simulink model "test"  (R2017b)
settings: Solver=FixedStepAuto  StartTime=0.0  StopTime=Tend  RelTol=1e-3  EnableMultiTasking=on
StartFcn:
  | params
values from neighbouring files (symbols this model uses):
  Tend = 30    [params.m]    (also in readingVoltage.m = 10)
  Ts = 0.01    [params.m]    (also in readingVoltage.m = 0.1)
libraries: arduinolib x4, cstblocks x1
settings Model: SimulationMode=external  ExtModeTrigDuration=2  Creator=s-tsujii  LastModifiedBy=s-tsujii
settings OptimizationCC: PassReuseOutputArgsThreshold=0  MaxStackSize=64
settings DebuggingCC: ParameterTunabilityLossMsg=error
settings HardwareCC: ProdBitPerInt=16  ProdBitPerPointer=16  ProdBitPerSizeT=16  ProdBitPerPtrDiffT=16  ProdLargestAtomicFloat=None  ProdWordSize=8  ProdHWDeviceType=Atmel->AVR  UseEmbeddedCoderFeatures=off  UseSimulinkCoderFeatures=off
settings SFSimCC: MATLABDynamicMemAlloc=off
settings RTWCC: SystemTargetFile=ert.tlc  HardwareBoard=Arduino Uno  TLCOptions=-aInlineSetEventsForThisBaseRateFcn=TLC_FALSE -aSuppressMultiTaskScheduler=TLC_FALSE -aRateBasedStepFcn=1  TemplateMakefile=ert_default_tmf  GenerateReport=on  Toolchain=Arduino AVR  BuildConfiguration=Faster Runs  LaunchReport=on
settings CodeAppCC: ForceParamTrailComments=on  OperatorAnnotations=on  MangleLength=10
settings ERTTargetCC: ERTCustomFileBanners=off  SupportContinuousTime=on  SupportNonInlinedSFcns=on  RemoveResetFunc=off  SupportVariableSizeSignals=on  ModelStepFunctionPrototypeControlCompliant=off

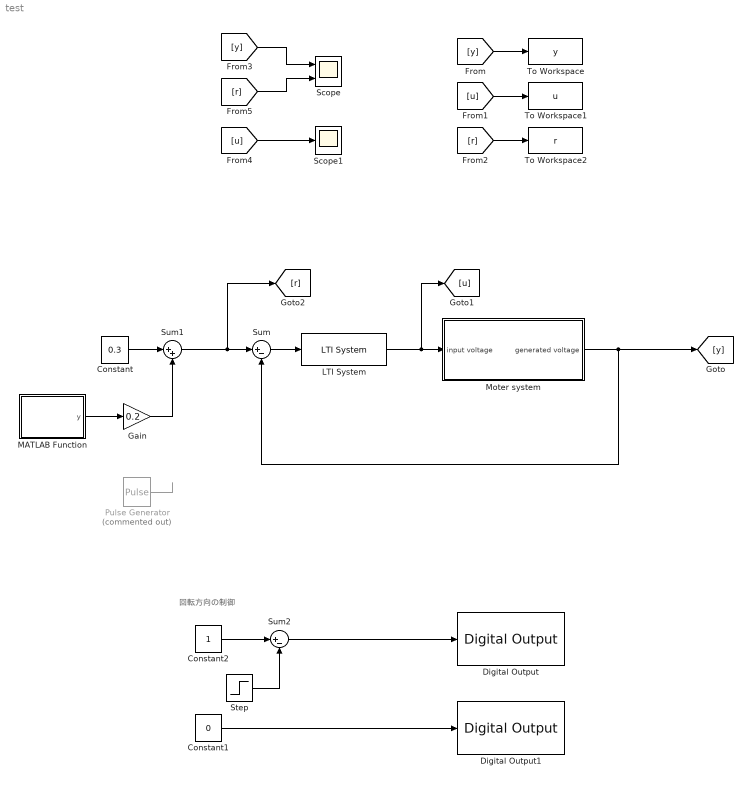
== system test ==
  note: 回転方向の制御
  Constant : Constant  Value=0.3
  Constant1 : Constant  Value=0
  Constant2 : Constant
  Digital Output : arduinolib/Digital Output  pinNumber=6  blockPlatform=arduino
  Digital Output1 : arduinolib/Digital Output  pinNumber=7  blockPlatform=arduino
  Gain : Gain  Gain=0.2
  LTI System : cstblocks/LTI System  sys=Cfb  IC=[]
  MATLAB Function : MATLAB Function  TreatAsAtomicUnit=on
  Moter system : Subsystem
  Pulse Generator : DiscretePulseGenerator  Commented=on  Amplitude=0.5  Period=4/Ts  PulseWidth=0.5*4/Ts  SampleTime=Ts
  Scope : Scope  NumInputPorts=2
  Scope1 : Scope
  Step : Step  Time=Tend-Ts  SampleTime=Ts
  Sum : Sum  Inputs=|+-
  Sum1 : Sum  Inputs=|++
  Sum2 : Sum  Inputs=|+-
  To Workspace : ToWorkspace  VariableName=y  SaveFormat=Structure With Time  SampleTime=-1
  To Workspace1 : ToWorkspace  VariableName=u  SaveFormat=Structure With Time  SampleTime=-1
  To Workspace2 : ToWorkspace  VariableName=r  SaveFormat=Structure With Time  SampleTime=-1
  wires:
  Sum/1 -> LTI System/1
  Sum1/1 -> [r], Sum/1
  Pulse Generator/1 -> ?
  Constant/1 -> Sum1/1
  Sum2/1 -> Digital Output/1
  Constant1/1 -> Digital Output1/1
  Constant2/1 -> Sum2/1
  Step/1 -> Sum2/2
  Moter system/1(generated voltage) -> Sum/2, [y]
  [y] -> To Workspace/1
  LTI System/1 -> [u], Moter system/1(input voltage)
  [u] -> To Workspace1/1
  [r] -> To Workspace2/1
  [y] -> Scope/1
  [r] -> Scope/2
  [u] -> Scope1/1
  Gain/1 -> Sum1/2
  MATLAB Function/1(y) -> Gain/1

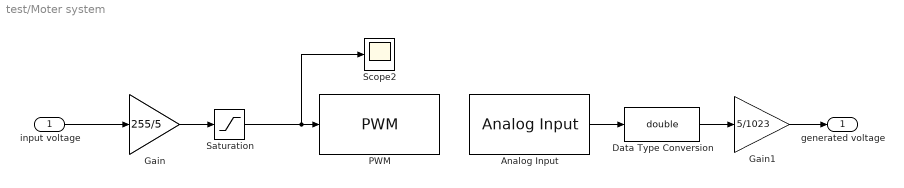
== system test/Moter system ==
  input voltage : Inport
  Analog Input : arduinolib/Analog Input  pinNumber=0  sampleTime=Ts  blockPlatform=arduino
  Data Type Conversion : DataTypeConversion  OutDataTypeStr=double
  Gain : Gain  Gain=255/5
  Gain1 : Gain  Gain=5/1023
  PWM : arduinolib/PWM  pinNumber=5  blockPlatform=arduino
  Saturation : Saturate  UpperLimit=255
  Scope2 : Scope
  generated voltage : Outport
  wires:
  Analog Input/1 -> Data Type Conversion/1
  Saturation/1 -> PWM/1, Scope2/1
  Gain1/1 -> generated voltage/1
  Data Type Conversion/1 -> Gain1/1
  input voltage/1 -> Gain/1
  Gain/1 -> Saturation/1

== matlab function test/MATLAB Function ==
  data: y output
function y = fcn()
% idinput 互換のPRBS(M系列)信号を生成する

persistent x;   % レジスタの状態
n = 10;         % レジスタの個数（段数）
p = [3,10];     % 生成多項式

if isempty(x)
    x = ones([n, 1]);   % 初期状態
end

y = 1 - 2*x(end);               % レジスタ値を出力

x0 = xor(x(p(1)), x(p(2)));     % 生成多項式によって新しい状態を作成
x = circshift(x, 1);            % レジスタの状態を更新
x(1) = x0;                      % 新しい状態を保存
end
